simulink model "hiv_model_ekf_loesung"  (R2019b)
settings: Solver=VariableStepAuto  StartTime=0.0  StopTime=20  RelTol=1e-6
values from neighbouring files (symbols this model uses):
  Delta = 1    [beispielsystem.m]    (also in init.m; init_loesung.m = 0.01; model_dsc.m = block.DialogPrm(1).data)
  P_0 = diag([(xdash0*pp).^2;(Theta*pp).^2])    [init_loesung.m]
  Theta = [0.25 50 0.25 10 0.01 0.0045]'    [init_loesung.m]
  W = zeros(9,9)    [init_loesung.m]
  x_hat_0 = [xdash_hat_0;Theta_hat_0]    [init_loesung.m]
  xdash0 = [1000 550 0.0001]'    [init_loesung.m]
  xdash12RL = [1000 550]'    [init_loesung.m]
  Z = diag([100,100,10^-5])    [init_loesung.m]
settings Model: Creator=schauer  LastModifiedBy=schauer

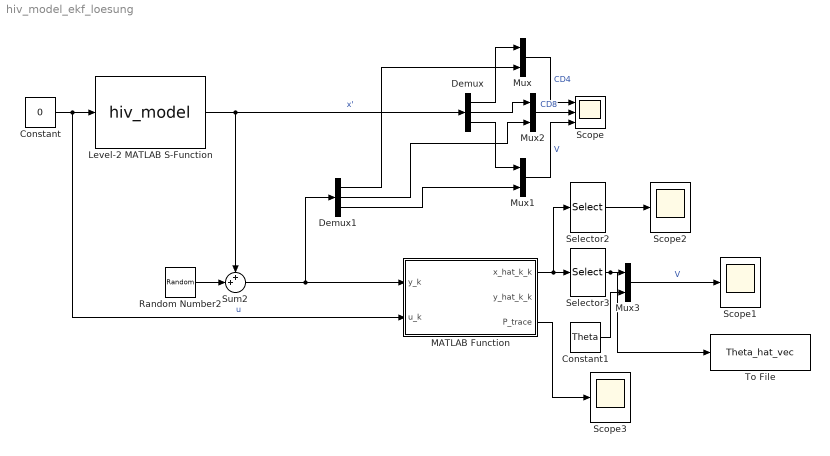
== system hiv_model_ekf_loesung ==
  Constant : Constant  Value=0
  Constant1 : Constant  Value=Theta
  Demux : Demux  Outputs=3
  Demux1 : Demux  Outputs=3
  Level-2 MATLAB S-Function : M-S-Function  FunctionName=hiv_model  Parameters=xdash0,Theta,xdash12RL
  MATLAB Function : MATLAB Function  TreatAsAtomicUnit=on  SystemSampleTime=Delta
  Mux{,1..3} (4 alike) : Mux  Inputs=2
  Random Number2 : RandomNumber  Variance=[100 100 10^-5]  SampleTime=Delta
  Scope : Scope  NumInputPorts=3
  Scope1 : Scope
  Scope2 : Scope
  Scope3 : Scope
  Selector2 : Selector  InputPortWidth=9  IndexOptions=Index vector (dialog)  Indices=[1:3]  OutputSizes=1
  Selector3 : Selector  InputPortWidth=9  IndexOptions=Index vector (dialog)  Indices=[4:9]  OutputSizes=1
  Sum2 : Sum  Inputs=++|
  To File : ToFile  Filename=Theta_hat_vec  MatrixName=Theta_hat_vec
  wires:
  Constant/1 -> MATLAB Function/2(u_k), Level-2 MATLAB S-Function/1  "u"
  Level-2 MATLAB S-Function/1 -> Demux/1, Sum2/1  "x'"
  Mux/1 -> Scope/1  "CD4"
  Demux/1 -> Mux/1
  Demux/3 -> Mux1/1
  Mux1/1 -> Scope/3  "V"
  Sum2/1 -> Demux1/1, MATLAB Function/1(y_k)
  MATLAB Function/1(x_hat_k_k) -> Selector2/1, Selector3/1
  Selector2/1 -> Scope2/1
  Mux3/1 -> Scope1/1  "V"
  Selector3/1 -> To File/1, Mux3/1
  Constant1/1 -> Mux3/2
  Random Number2/1 -> Sum2/2
  Mux2/1 -> Scope/2  "CD8"
  Demux/2 -> Mux2/1
  Demux1/1 -> Mux/2
  Demux1/2 -> Mux2/2
  Demux1/3 -> Mux1/2
  MATLAB Function/3(P_trace) -> Scope3/1

== matlab function hiv_model_ekf_loesung/MATLAB Function ==
  data: y_k input; x_hat_k_k output; u_k input; x_hat_0 parameter; P_0 parameter; y_hat_k_k output; P_trace output; W parameter; Z parameter; xdash12RL parameter; Delta parameter
function [x_hat_k_k,y_hat_k_k,P_trace] = fcn(y_k,u_k,x_hat_0,P_0,W,Z,xdash12RL,Delta)
%initialize states (variables to be stored)
persistent  x_hat_k_km1 P_k_km1;
if isempty( x_hat_k_km1) 
    x_hat_k_km1=x_hat_0;
end
if isempty( P_k_km1)
    P_k_km1=P_0;
end
%Update 
C_km1 = [1 0 0 0 0 0 0 0 0
         0 1 0 0 0 0 0 0 0
         0 0 1 0 0 0 0 0 0];
K_k=P_k_km1*C_km1'*inv(Z+C_km1*P_k_km1*C_km1');
x_hat_k_k=x_hat_k_km1+K_k*(y_k-C_km1*x_hat_k_km1);
P_k_k=P_k_km1-K_k*C_km1*P_k_km1;
%Linearisation
A_k=zeros(9,9);
A_k(1,1)=1+Delta*(-x_hat_k_k(4)-x_hat_k_k(5)*x_hat_k_k(3));
A_k(1,3)=Delta*(-x_hat_k_k(5)*x_hat_k_k(1)); 
A_k(1,4)=Delta*(-x_hat_k_k(1)+xdash12RL(1));
A_k(1,5)=Delta*(-x_hat_k_k(1)*x_hat_k_k(3));
A_k(2,2)=1+Delta*(-x_hat_k_k(6)+x_hat_k_k(7)*x_hat_k_k(3));
A_k(2,3)=Delta*(x_hat_k_k(7)*x_hat_k_k(2));
A_k(2,6)=Delta*(-x_hat_k_k(2)+xdash12RL(2));
A_k(2,7)=Delta*(+x_hat_k_k(2)*x_hat_k_k(3));
A_k(3,1)=Delta*(+x_hat_k_k(8)*x_hat_k_k(3));
A_k(3,2)=Delta*(-x_hat_k_k(9)*x_hat_k_k(3));
A_k(3,3)=1+Delta*(+x_hat_k_k(8)*x_hat_k_k(1)-...
    x_hat_k_k(9)*x_hat_k_k(2));
A_k(3,8)=Delta*(+x_hat_k_k(1)*x_hat_k_k(3));
A_k(3,9)=Delta*(-x_hat_k_k(2)*x_hat_k_k(3));
A_k(4:9,4:9)=eye(6,6);
%B_k=[0 0 -1 0 0 0 0 0 0]';
%Prediction
P_kp1_k=A_k*P_k_k*A_k'+W;
x_hat_kp1_k=[x_hat_k_k(1)+Delta*(-x_hat_k_k(4)*x_hat_k_k(1)-...
       x_hat_k_k(5)*x_hat_k_k(1)*x_hat_k_k(3)+...
       x_hat_k_k(4)*xdash12RL(1));
     x_hat_k_k(2)+Delta*(-x_hat_k_k(6)*x_hat_k_k(2)+...
             x_hat_k_k(7)*x_hat_k_k(2)*x_hat_k_k(3)+...
             x_hat_k_k(6)*xdash12RL(2));
     x_hat_k_k(3)+Delta*(x_hat_k_k(8)*x_hat_k_k(1)*...
             x_hat_k_k(3)-x_hat_k_k(9)*x_hat_k_k(2)*...
             x_hat_k_k(3)-u_k);
     x_hat_k_k(4:9)];     
%y_hat(k|k)
C_k=C_km1;
y_hat_k_k=C_k*x_hat_k_k;
P_trace=trace(P_k_k);
%Store states
P_k_km1=P_kp1_k;
x_hat_k_km1=x_hat_kp1_k;
